simulink model "cartesianController"  (R2012b)
settings: Solver=ode45  StartTime=0.0  StopTime=30  RelTol=1e-3
libraries: dspmtrx3 x8
settings Model: Creator=aruszkowski  LastModifiedBy=davinci
settings DataIOCC: SignalLoggingSaveFormat=ModelDataLogs  SaveOutput=off  SaveTime=off
settings OptimizationCC: ExpressionDepthLimit=128
settings DebuggingCC: ReadBeforeWriteMsg=DisableAll  WriteAfterWriteMsg=DisableAll  WriteAfterReadMsg=DisableAll  MultiTaskDSMMsg=warning  MultiTaskCondExecSysMsg=none  StateNameClashWarn=none  StrictBusMsg=None
settings ModelReferenceCC: UpdateModelReferenceTargets=IfOutOfDate
settings SFSimCC: SFSimEcho=off
settings RTWCC: IncludeERTFirstTime=on
settings CodeAppCC: CustomSymbolStrType=$N$R$M_T  InternalIdentifier=Shortened

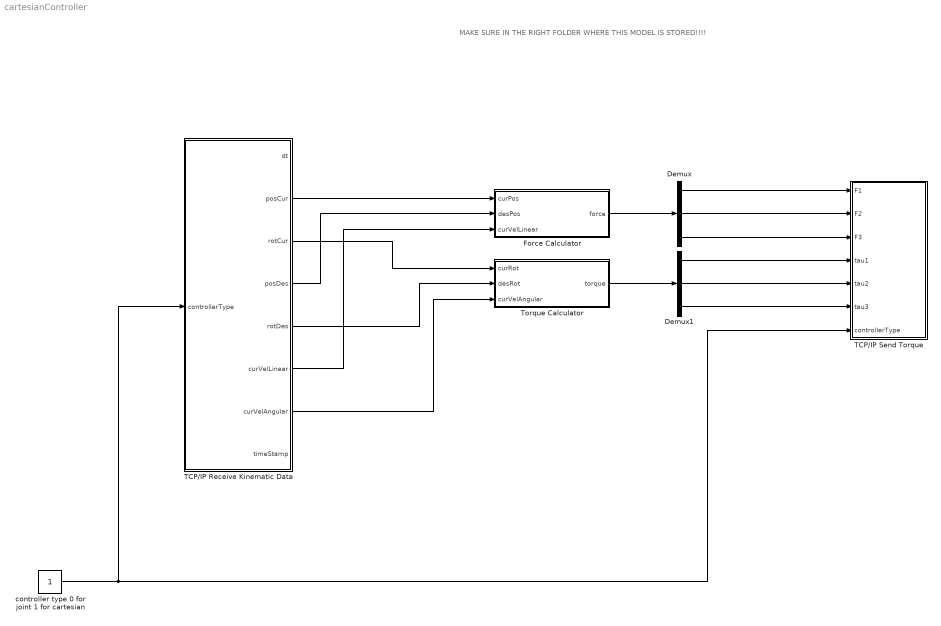
== system cartesianController ==
  note: MAKE SURE IN THE RIGHT FOLDER WHERE THIS MODEL IS STORED!!!!
  Demux : Demux  Outputs=3
  Demux1 : Demux  Outputs=3
  Force Calculator : Subsystem
  TCP/IP Receive Kinematic Data : Subsystem
  TCP/IP Send Torque : Subsystem  TreatAsAtomicUnit=on
  Torque Calculator : Subsystem
  controller type 0 for joint 1 for cartesian : Constant
  wires:
  controller type 0 for joint 1 for cartesian/1 -> TCP/IP Receive Kinematic Data/1(controllerType), TCP/IP Send Torque/7(controllerType)
  Force Calculator/1(force) -> Demux/1
  Demux/1 -> TCP/IP Send Torque/1(F1)
  Demux/2 -> TCP/IP Send Torque/2(F2)
  Demux/3 -> TCP/IP Send Torque/3(F3)
  Torque Calculator/1(torque) -> Demux1/1
  Demux1/1 -> TCP/IP Send Torque/4(tau1)
  Demux1/2 -> TCP/IP Send Torque/5(tau2)
  Demux1/3 -> TCP/IP Send Torque/6(tau3)
  TCP/IP Receive Kinematic Data/2(posCur) -> Force Calculator/1(curPos)
  TCP/IP Receive Kinematic Data/4(posDes) -> Force Calculator/2(desPos)
  TCP/IP Receive Kinematic Data/6(curVelLinear) -> Force Calculator/3(curVelLinear)
  TCP/IP Receive Kinematic Data/3(rotCur) -> Torque Calculator/1(curRot)
  TCP/IP Receive Kinematic Data/5(rotDes) -> Torque Calculator/2(desRot)
  TCP/IP Receive Kinematic Data/7(curVelAngular) -> Torque Calculator/3(curVelAngular)

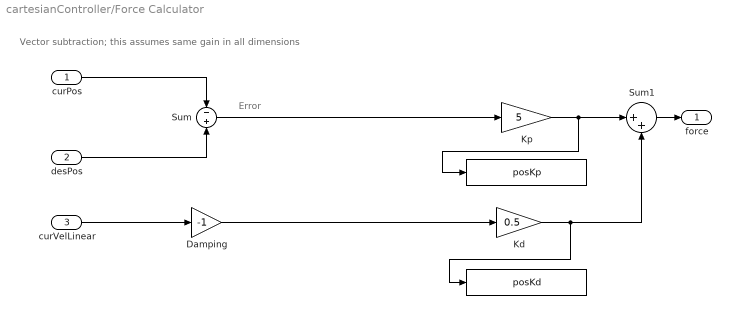
== system cartesianController/Force Calculator ==
  note: Vector subtraction;
      | this assumes same gain in all dimensions
  note: Error
  curPos : Inport
  desPos : Inport  Port=2
  curVelLinear : Inport  Port=3
  "      " : ToWorkspace  VariableName=posKp  SampleTime=-1  SaveFormat=Timeseries
  "        " : ToWorkspace  VariableName=posKd  SampleTime=-1  SaveFormat=Timeseries
  Damping : Gain  Gain=-1
  Kd : Gain  Gain=0.5
  Kp : Gain  Gain=5
  Sum : Sum  Inputs=-|+
  Sum1 : Sum  Inputs=|++
  force : Outport
  wires:
  Kp/1 -> Sum1/1, "      "/1
  Kd/1 -> Sum1/2, "        "/1
  Sum1/1 -> force/1
  curVelLinear/1 -> Damping/1
  Damping/1 -> Kd/1
  Sum/1 -> Kp/1
  desPos/1 -> Sum/2
  curPos/1 -> Sum/1

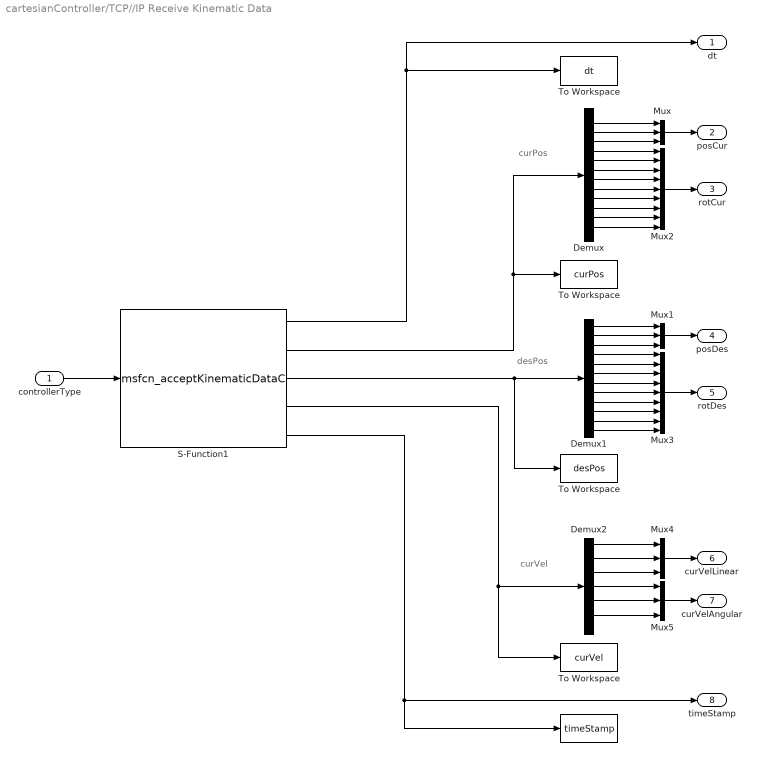
== system cartesianController/TCP//IP Receive Kinematic Data ==
  note: curVel
  note: desPos
  note: curPos
  controllerType : Inport
  " " : ToWorkspace  VariableName=timeStamp  SampleTime=-1  SaveFormat=Timeseries
  Demux : Demux  Outputs=12
  Demux1 : Demux  Outputs=12
  Demux2 : Demux  Outputs=7
  Mux{,1,4..5} (4 alike) : Mux  Inputs=3
  Mux2 : Mux  Inputs=9
  Mux3 : Mux  Inputs=9
  S-Function1 : S-Function  FunctionName=msfcn_acceptKinematicDataC  Parameters='137.82.56.245', '12345'  EnableBusSupport=off
  To Workspace : ToWorkspace  VariableName=curPos  SampleTime=-1  SaveFormat=Timeseries
  "To Workspace " : ToWorkspace  VariableName=desPos  SampleTime=-1  SaveFormat=Timeseries
  "To Workspace " : ToWorkspace  VariableName=curVel  SampleTime=-1  SaveFormat=Timeseries
  "To Workspace " : ToWorkspace  VariableName=dt  SampleTime=-1  SaveFormat=Timeseries
  dt : Outport
  posCur : Outport  Port=2
  rotCur : Outport  Port=3
  posDes : Outport  Port=4
  rotDes : Outport  Port=5
  curVelLinear : Outport  Port=6
  curVelAngular : Outport  Port=7
  timeStamp : Outport  Port=8
  wires:
  S-Function1/1 -> "To Workspace "/1, dt/1
  S-Function1/4 -> "To Workspace "/1, Demux2/1
  S-Function1/3 -> "To Workspace "/1, Demux1/1
  S-Function1/2 -> To Workspace/1, Demux/1
  S-Function1/5 -> " "/1, timeStamp/1
  controllerType/1 -> S-Function1/1
  Demux/1 -> Mux/1
  Demux/2 -> Mux/2
  Demux/3 -> Mux/3
  Mux/1 -> posCur/1
  Demux1/1 -> Mux1/1
  Demux1/2 -> Mux1/2
  Demux1/3 -> Mux1/3
  Mux1/1 -> posDes/1
  Demux/4 -> Mux2/1
  Demux/5 -> Mux2/2
  Demux/6 -> Mux2/3
  Demux/7 -> Mux2/4
  Demux/8 -> Mux2/5
  Demux/9 -> Mux2/6
  Demux/10 -> Mux2/7
  Demux/11 -> Mux2/8
  Demux/12 -> Mux2/9
  Mux2/1 -> rotCur/1
  Demux1/6 -> Mux3/3
  Demux1/7 -> Mux3/4
  Demux1/8 -> Mux3/5
  Demux1/9 -> Mux3/6
  Demux1/10 -> Mux3/7
  Demux1/11 -> Mux3/8
  Demux1/12 -> Mux3/9
  Mux3/1 -> rotDes/1
  Demux1/5 -> Mux3/2
  Demux1/4 -> Mux3/1
  Mux4/1 -> curVelLinear/1
  Demux2/1 -> Mux4/1
  Demux2/2 -> Mux4/2
  Demux2/3 -> Mux4/3
  Demux2/4 -> Mux5/1
  Demux2/5 -> Mux5/2
  Demux2/6 -> Mux5/3
  Mux5/1 -> curVelAngular/1

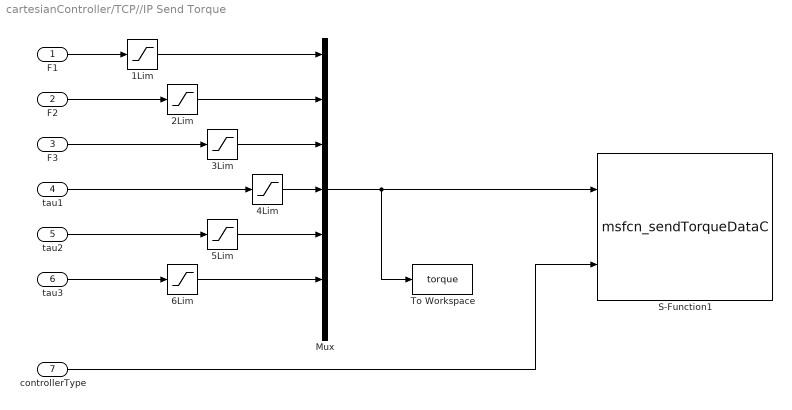
== system cartesianController/TCP//IP Send Torque ==
  F1 : Inport
  F2 : Inport  Port=2
  F3 : Inport  Port=3
  tau1 : Inport  Port=4
  tau2 : Inport  Port=5
  tau3 : Inport  Port=6
  controllerType : Inport  Port=7
  1Lim : Saturate  UpperLimit=900  LowerLimit=-900
  2Lim : Saturate  UpperLimit=900  LowerLimit=-900
  3Lim : Saturate  UpperLimit=900  LowerLimit=-900
  4Lim : Saturate  UpperLimit=900  LowerLimit=-900
  5Lim : Saturate  UpperLimit=900  LowerLimit=-900
  6Lim : Saturate  UpperLimit=900  LowerLimit=-900
  Mux : Mux  Inputs=7
  S-Function1 : S-Function  FunctionName=msfcn_sendTorqueDataC  Parameters='137.82.56.245', '54321'  EnableBusSupport=off
  To Workspace : ToWorkspace  VariableName=torque  SampleTime=-1  SaveFormat=Timeseries
  wires:
  Mux/1 -> S-Function1/1, To Workspace/1
  tau3/1 -> 6Lim/1
  tau2/1 -> 5Lim/1
  tau1/1 -> 4Lim/1
  F3/1 -> 3Lim/1
  F2/1 -> 2Lim/1
  F1/1 -> 1Lim/1
  1Lim/1 -> Mux/1
  2Lim/1 -> Mux/2
  3Lim/1 -> Mux/3
  5Lim/1 -> Mux/5
  6Lim/1 -> Mux/6
  4Lim/1 -> Mux/4
  controllerType/1 -> S-Function1/2

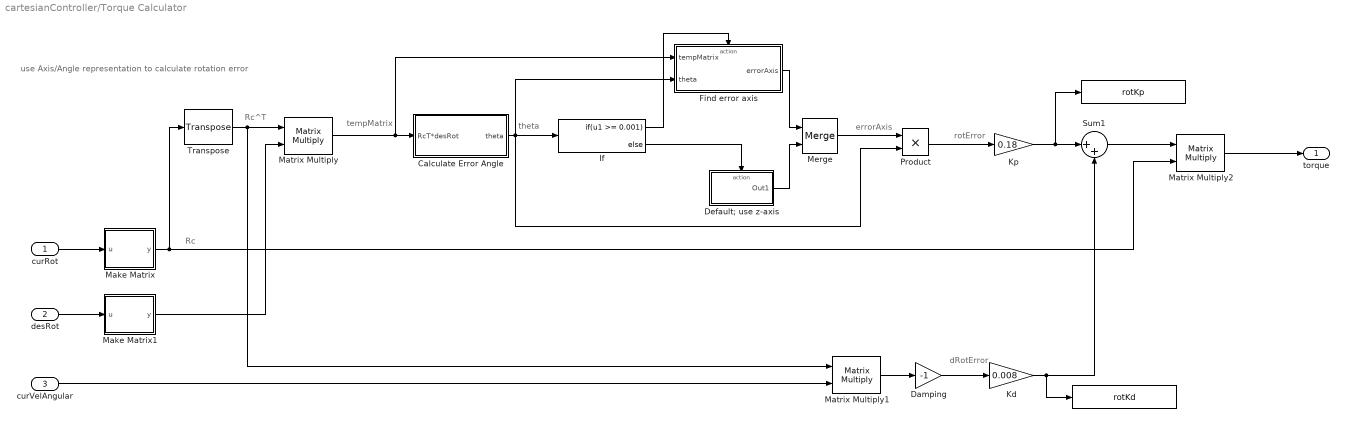
== system cartesianController/Torque Calculator ==
  note: dRotError
  note: rotError
  note: errorAxis
  note: use Axis/Angle representation to calculate rotation error
  note: theta
  note: tempMatrix
  note: Rc^T
  note: Rc
  curRot : Inport
  desRot : Inport  Port=2
  curVelAngular : Inport  Port=3
  "      " : ToWorkspace  VariableName=rotKp  SampleTime=-1  SaveFormat=Timeseries
  "        " : ToWorkspace  VariableName=rotKd  SampleTime=-1  SaveFormat=Timeseries
  Calculate Error Angle : Subsystem
  Damping : Gain  Gain=-1
  Default; use z-axis : Subsystem  TreatAsAtomicUnit=on
  Find error axis : Subsystem  TreatAsAtomicUnit=on
  If : If  IfExpression=u1 >= 0.001
  Kd : Gain  Gain=0.008
  Kp : Gain  Gain=0.18
  Make Matrix : MATLAB Function  TreatAsAtomicUnit=on
  Make Matrix1 : MATLAB Function  TreatAsAtomicUnit=on
  Matrix Multiply : Product  Multiplication=Matrix(*)
  Matrix Multiply1 : Product  Multiplication=Matrix(*)
  Matrix Multiply2 : Product  Multiplication=Matrix(*)
  Merge : Merge
  Product : Product  RndMeth=Zero
  Sum1 : Sum  Inputs=|++
  Transpose : dspmtrx3/Transpose  Hermitian=off  overflowFlag=off
  torque : Outport
  wires:
  Kp/1 -> "      "/1, Sum1/1
  Kd/1 -> Sum1/2, "        "/1
  Damping/1 -> Kd/1
  curRot/1 -> Make Matrix/1(u)
  Make Matrix/1(y) -> Matrix Multiply2/2, Transpose/1
  desRot/1 -> Make Matrix1/1(u)
  Make Matrix1/1(y) -> Matrix Multiply/2
  Transpose/1 -> Matrix Multiply/1, Matrix Multiply1/1
  If/2 -> Default; use z-axis/Action
  If/1 -> Find error axis/Action
  Find error axis/1(errorAxis) -> Merge/1
  Default; use z-axis/1(Out1) -> Merge/2
  Merge/1 -> Product/1
  Calculate Error Angle/1(theta) -> Find error axis/2(theta), Product/2, If/1
  Matrix Multiply/1 -> Find error axis/1(tempMatrix), Calculate Error Angle/1(RcT*desRot)
  Product/1 -> Kp/1
  Matrix Multiply1/1 -> Damping/1
  Sum1/1 -> Matrix Multiply2/1
  Matrix Multiply2/1 -> torque/1
  curVelAngular/1 -> Matrix Multiply1/2

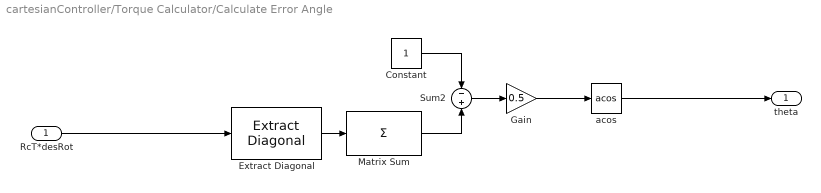
== system cartesianController/Torque Calculator/Calculate Error Angle ==
  RcT*desRot : Inport
  Constant : Constant
  Extract Diagonal : dspmtrx3/Extract Diagonal
  Gain : Gain  Gain=0.5
  Matrix Sum : Sum  Inputs=+
  Sum2 : Sum  Inputs=-|+
  acos : Trigonometry  Operator=acos
  theta : Outport
  wires:
  RcT*desRot/1 -> Extract Diagonal/1
  Sum2/1 -> Gain/1
  Gain/1 -> acos/1
  Constant/1 -> Sum2/1
  Extract Diagonal/1 -> Matrix Sum/1
  Matrix Sum/1 -> Sum2/2
  acos/1 -> theta/1

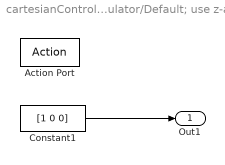
== system cartesianController/Torque Calculator/Default; use z-axis ==
  Action Port : ActionPort  ActionType=else
  Constant1 : Constant  Value=[1 0 0]
  Out1 : Outport  InitialOutput=[1 0 0]
  wires:
  Constant1/1 -> Out1/1

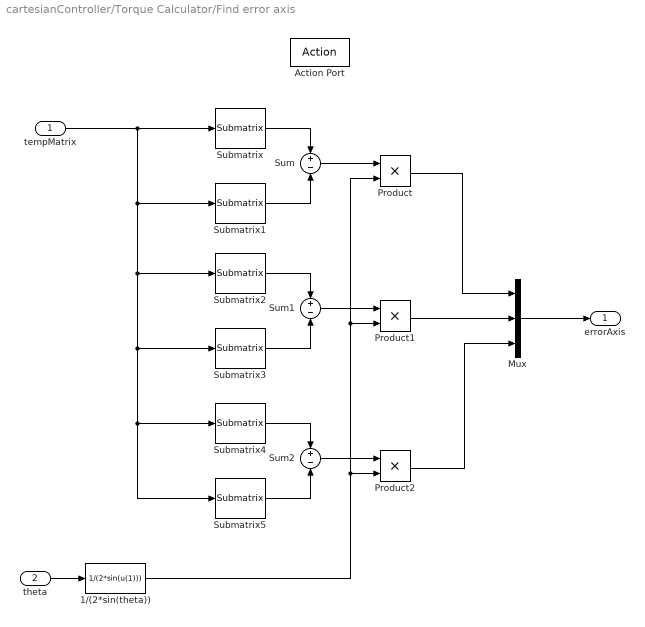
== system cartesianController/Torque Calculator/Find error axis ==
  tempMatrix : Inport
  theta : Inport  Port=2
  Action Port : ActionPort  ActionType=then
  1/(2*sin(theta)) : Fcn  Expr=1/(2*sin(u(1)))
  Mux : Mux  Inputs=3
  Product : Product  RndMeth=Zero
  Product1 : Product  RndMeth=Zero
  Product2 : Product  RndMeth=Zero
  Submatrix : dspmtrx3/Submatrix  RowSpan=One row  RowStartMode=Last  RowStartIndex=1  RowEndMode=Last  RowEndIndex=1  ColSpan=One column  ColStartMode=Middle  ColStartIndex=1  ColEndMode=Last  ColEndIndex=1
  Submatrix1 : dspmtrx3/Submatrix  RowSpan=One row  RowStartMode=Middle  RowStartIndex=1  RowEndMode=Last  RowEndIndex=1  ColSpan=One column  ColStartMode=Last  ColStartIndex=1  ColEndMode=Last  ColEndIndex=1
  Submatrix2 : dspmtrx3/Submatrix  RowSpan=One row  RowStartMode=First  RowStartIndex=1  RowEndMode=Last  RowEndIndex=1  ColSpan=One column  ColStartMode=Last  ColStartIndex=1  ColEndMode=Last  ColEndIndex=1
  Submatrix3 : dspmtrx3/Submatrix  RowSpan=One row  RowStartMode=Last  RowStartIndex=1  RowEndMode=Last  RowEndIndex=1  ColSpan=One column  ColStartMode=First  ColStartIndex=1  ColEndMode=Last  ColEndIndex=1
  Submatrix4 : dspmtrx3/Submatrix  RowSpan=One row  RowStartMode=Middle  RowStartIndex=1  RowEndMode=Last  RowEndIndex=1  ColSpan=One column  ColStartMode=First  ColStartIndex=1  ColEndMode=Last  ColEndIndex=1
  Submatrix5 : dspmtrx3/Submatrix  RowSpan=One row  RowStartMode=First  RowStartIndex=1  RowEndMode=Last  RowEndIndex=1  ColSpan=One column  ColStartMode=Middle  ColStartIndex=1  ColEndMode=Last  ColEndIndex=1
  Sum : Sum  Inputs=+|-
  Sum1 : Sum  Inputs=+|-
  Sum2 : Sum  Inputs=+|-
  errorAxis : Outport
  wires:
  theta/1 -> 1/(2*sin(theta))/1
  tempMatrix/1 -> Submatrix1/1, Submatrix2/1, Submatrix3/1, Submatrix4/1, Submatrix5/1, Submatrix/1
  Submatrix/1 -> Sum/1
  Submatrix1/1 -> Sum/2
  Submatrix2/1 -> Sum1/1
  Submatrix3/1 -> Sum1/2
  Submatrix4/1 -> Sum2/1
  Submatrix5/1 -> Sum2/2
  1/(2*sin(theta))/1 -> Product2/2, Product/2, Product1/2
  Sum/1 -> Product/1
  Sum2/1 -> Product2/1
  Sum1/1 -> Product1/1
  Product/1 -> Mux/1
  Product1/1 -> Mux/2
  Product2/1 -> Mux/3
  Mux/1 -> errorAxis/1

== matlab function cartesianController/Torque Calculator/Make Matrix1 ==
  data: u input; y output
function y = fcn(u)
%#codegen

y = [u(1) u(2) u(3); u(4) u(5) u(6); u(7) u(8) u(9)]

== matlab function cartesianController/Torque Calculator/Make Matrix ==
  data: u input; y output
function y = fcn(u)
%#codegen

y = [u(1) u(2) u(3); u(4) u(5) u(6); u(7) u(8) u(9)]
